simulink model "T1"  (R2025a)
settings: Solver=FixedStepDiscrete  StartTime=0.0  StopTime=1  FixedStep=Auto  RelTol=1e-3
libraries: hwlogiciolib x1
settings Model: Creator=mahij  LastModifiedBy=mahij

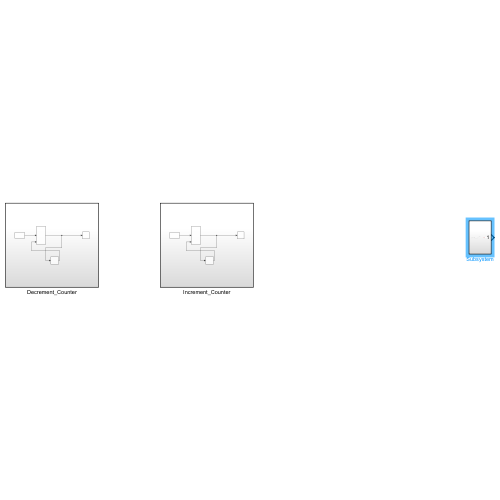
[thumbnail: Simulink's stored preview of the top-level diagram]
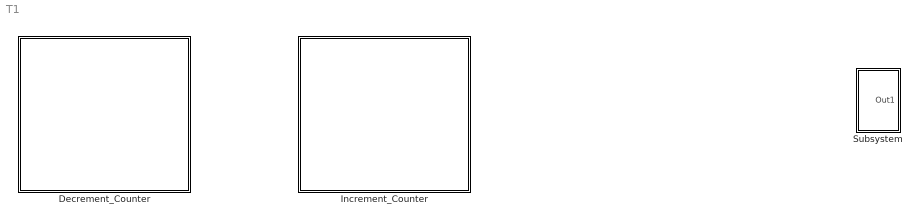
== system T1 ==
  Decrement_Counter : Subsystem
  Increment_Counter : Subsystem
  Subsystem : Subsystem

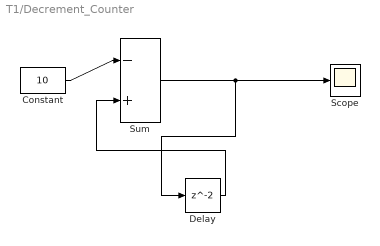
== system T1/Decrement_Counter ==
  Constant : Constant  Value=10
  Delay : Delay
  Scope : Scope
      settings: ActiveDisplayYMinimum=-2822.5  ActiveDisplayYMaximum=302.49999999999994
  Sum : Sum  Inputs=|-+
  wires:
  Delay/1 -> Sum/2
  Sum/1 -> Delay/1, Scope/1
  Constant/1 -> Sum/1

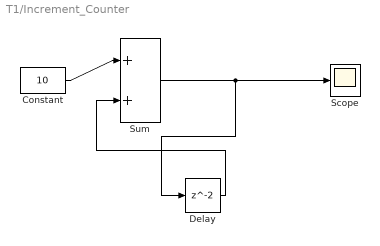
== system T1/Increment_Counter ==
  Constant : Constant  Value=10
  Delay : Delay
  Scope : Scope
      settings: ActiveDisplayYMinimum=-2822.5  ActiveDisplayYMaximum=302.49999999999994
  Sum : Sum  Inputs=|++
  wires:
  Delay/1 -> Sum/2
  Sum/1 -> Delay/1, Scope/1
  Constant/1 -> Sum/1

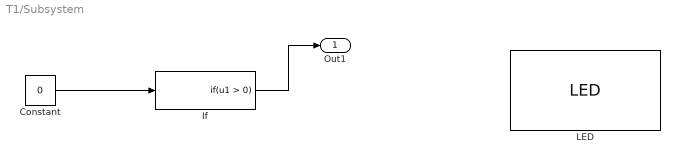
== system T1/Subsystem ==
  Constant : Constant  Value=0
  If : If  ShowElse=off
  LED : hwlogiciolib/LED  NumLeds=1  LastTargetBoard=None  MaxNumLeds=24
  Out1 : Outport
  wires:
  If/1 -> Out1/1
  Constant/1 -> If/1
  ? -> LED/1
